simulink model "Modele_MCC_v2017a"  (R2017a)
settings: Solver=ode45  StartTime=0.0  StopTime=10  RelTol=1e-6  AbsTol=1e-6
values from neighbouring files (symbols this model uses):
  f = 1e-1    (= 0.1)    [Initialisation_MCC.m]
  J = 1e-2    (= 0.01)    [Initialisation_MCC.m]
  k = 0.05    [Initialisation_MCC.m]
  L = 1e-1    (= 0.1)    [Initialisation_MCC.m]
  R = 50    [Initialisation_MCC.m]
settings Model: Creator=Alexis  LastModifiedBy=Alexis
settings SolverCC: ShapePreserveControl=EnableAll  ZeroCrossAlgorithm=Adaptive

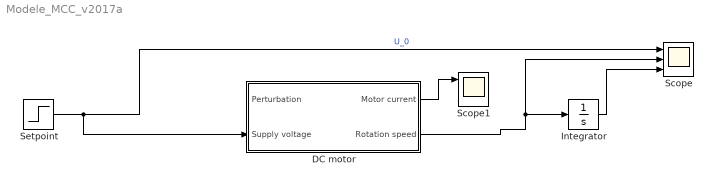
== system Modele_MCC_v2017a ==
  DC motor : Subsystem
  Integrator : Integrator
  Scope : Scope  NumInputPorts=3
  Scope1 : Scope  NumInputPorts=3
  Setpoint : Step  SampleTime=0
  wires:
  Setpoint/1 -> DC motor/2(Supply voltage), Scope/1  "U_0"
  Integrator/1 -> Scope/3
  DC motor/1(Motor current) -> Scope1/1
  DC motor/2(Rotation speed) -> Scope/2, Integrator/1

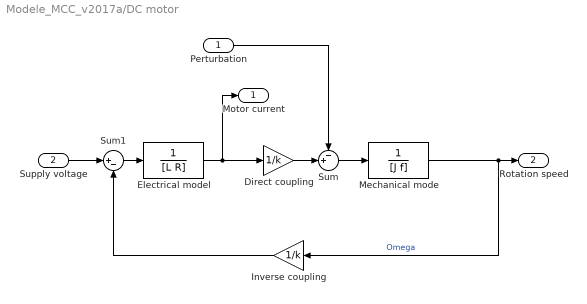
== system Modele_MCC_v2017a/DC motor ==
  Perturbation : Inport
  Supply voltage : Inport  Port=2
  Direct coupling : Gain  Gain=1/k
  Electrical model : TransferFcn  Denominator=[L R]
  Inverse coupling : Gain  Gain=1/k
  Mechanical mode : TransferFcn  Denominator=[J f]
  Sum : Sum  Inputs=-+|
  Sum1 : Sum  Inputs=|+-
  Motor current : Outport
  Rotation speed : Outport  Port=2
  wires:
  Direct coupling/1 -> Sum/2
  Sum/1 -> Mechanical mode/1
  Mechanical mode/1 -> Rotation speed/1, Inverse coupling/1  "Omega"
  Sum1/1 -> Electrical model/1
  Inverse coupling/1 -> Sum1/2
  Perturbation/1 -> Sum/1
  Supply voltage/1 -> Sum1/1
  Electrical model/1 -> Direct coupling/1, Motor current/1
